simulink library "Lib_AP_Math"  (R2014b)
settings: Solver=ode45  StartTime=0.0  StopTime=10.0  RelTol=1e-3
settings Model: Creator=Ehang  LastModifiedBy=Ehang

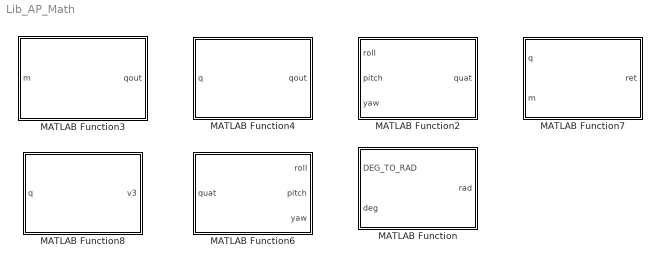
== system Lib_AP_Math ==
  MATLAB Function : MATLAB Function  TreatAsAtomicUnit=on
  MATLAB Function2 : MATLAB Function  TreatAsAtomicUnit=on
  MATLAB Function3 : MATLAB Function  TreatAsAtomicUnit=on
  MATLAB Function4 : MATLAB Function  TreatAsAtomicUnit=on
  MATLAB Function6 : MATLAB Function  TreatAsAtomicUnit=on
  MATLAB Function7 : MATLAB Function  TreatAsAtomicUnit=on
  MATLAB Function8 : MATLAB Function  TreatAsAtomicUnit=on

== matlab function Lib_AP_Math/MATLAB Function ==
  data: DEG_TO_RAD input; deg input; rad output
function rad = radians(DEG_TO_RAD,deg)
%#codegen
%将角度转化为弧度
rad = deg*DEG_TO_RAD;

== matlab function Lib_AP_Math/MATLAB Function2 ==
  data: roll input; pitch input; quat output; yaw input
function quat= from_euler(roll,pitch,yaw)
%%将欧拉角转化为四元数
%#codegen
    cr2 = cos(roll*0.5);
    cp2 = cos(pitch*0.5);
    cy2 = cos(yaw*0.5);
    sr2 = sin(roll*0.5);
    sp2 = sin(pitch*0.5);
    sy2 = sin(yaw*0.5);

    q1 = cr2*cp2*cy2 + sr2*sp2*sy2;
    q2 = sr2*cp2*cy2 - cr2*sp2*sy2;
    q3 = cr2*sp2*cy2 + sr2*cp2*sy2;
    q4 = cr2*cp2*sy2 - sr2*sp2*cy2;
    quat=[q1;q2;q3;q4];

% void Quaternion::from_euler(float roll, float pitch, float yaw)
% {
%     float cr2 = cosf(roll*0.5f);
%     float cp2 = cosf(pitch*0.5f);
%     float cy2 = cosf(yaw*0.5f);
%     float sr2 = sinf(roll*0.5f);
%     float sp2 = sinf(pitch*0.5f);
%     float sy2 = sinf(yaw*0.5f);
% 
%     q1 = cr2*cp2*cy2 + sr2*sp2*sy2;
%     q2 = sr2*cp2*cy2 - cr2*sp2*sy2;
%     q3 = cr2*sp2*cy2 + sr2*cp2*sy2;
%     q4 = cr2*cp2*sy2 - sr2*sp2*cy2;
% }

== matlab function Lib_AP_Math/MATLAB Function3 ==
  data: m input; qout output
function qout=from_rotation_matrix(m)
%#codegen
% //返回与旋转矩阵m等效的四元数qout
% // return the rotation matrix equivalent for this quaternion
% // Thanks to Martin John Baker
% // http://www.euclideanspace.com/maths/geometry/rotations/conversions/matrixToQuaternion/index.htm
%a,b,c是列数，x,y,z是行数
    m00 = m(1,1);
    m11 = m(2,2);
    m22 = m(3,3);
    m10 = m(1,2);
    m01 = m(2,1);
    m20 = m(1,3);
    m02 = m(3,1);
    m21 = m(2,3);
    m12 = m(3,2);
% m00 = m.a.x;
%     m11 = m.b.y;
%     m22 = m.c.z;
%     m10 = m.b.x;
%     m01 = m.a.y;
%     m20 = m.c.x;
%     m02 = m.a.z;
%     m21 = m.c.y;
%     m12 = m.b.z;
tr = m00 + m11 + m22;
%为什么有下划线 Matalb中elseif是连在一起的
    if (tr > 0) 
        S = sqrt(tr+1) * 2;
        qw = 0.25 * S;
        qx = (m21 - m12) / S;
        qy = (m02 - m20) / S;
        qz = (m10 - m01) / S;
    elseif (m00 > m11) && (m00 > m22) 
        S = sqrt(1.0 + m00 - m11 - m22) * 2;
        qw = (m21 - m12) / S;
        qx = 0.25 * S;
        qy = (m01 + m10) / S;
        qz = (m02 + m20) / S;
    elseif (m11 > m22) 
        S = sqrt(1.0+m11- m00 - m22) * 2;
        qw = (m02 - m20) / S;
        qx = (m01 + m10) / S;
        qy = 0.25* S;
        qz = (m12 + m21) / S;
    else 
        S = sqrt(1.0 + m22 - m00 - m11) * 2;
        qw = (m10 - m01) / S;
        qx = (m02 + m20) / S;
        qy = (m12 + m21) / S;
        qz = 0.25 * S;
    end
    qout=[qw;
          qx;
          qy;
          qz];

% // return the rotation matrix equivalent for this quaternion
% // Thanks to Martin John Baker
% // http://www.euclideanspace.com/maths/geometry/rotations/conversions/matrixToQuaternion/index.htm
% void Quaternion::from_rotation_matrix(const Matrix3f &m)
% {
%     const float &m00 = m.a.x;
%     const float &m11 = m.b.y;
%     const float &m22 = m.c.z;
%     const float &m10 = m.b.x;
%     const float &m01 = m.a.y;
%     const float &m20 = m.c.x;
%     const float &m02 = m.a.z;
%     const float &m21 = m.c.y;
%     const float &m12 = m.b.z;
%     float &qw = q1;
%     float &qx = q2;
%     float &qy = q3;
%     float &qz = q4;
% 
%     float tr = m00 + m11 + m22;
% 
%     if (tr > 0) {
%         float S = sqrtf(tr+1) * 2;
%         qw = 0.25f * S;
%         qx = (m21 - m12) / S;
%         qy = (m02 - m20) / S;
%         qz = (m10 - m01) / S;
%     } else if ((m00 > m11) && (m00 > m22)) {
%         float S = sqrtf(1.0f + m00 - m11 - m22) * 2;
%         qw = (m21 - m12) / S;
%         qx = 0.25f * S;
%         qy = (m01 + m10) / S;
%         qz = (m02 + m20) / S;
%     } else if (m11 > m22) {
%         float S = sqrtf(1.0f + m11 - m00 - m22) * 2;
%         qw = (m02 - m20) / S;
%         qx = (m01 + m10) / S;
%         qy = 0.25f * S;
%         qz = (m12 + m21) / S;
%     } else {
%         float S = sqrtf(1.0f + m22 - m00 - m11) * 2;
%         qw = (m10 - m01) / S;
%         qx = (m02 + m20) / S;
%         qy = (m12 + m21) / S;
%         qz = 0.25f * S;
%     }
% }

== matlab function Lib_AP_Math/MATLAB Function4 ==
  data: q input; qout output
function qout=inverse(q)
%#codegen
%四元素求逆
qout=[q(1), -q(2), -q(3), -q(4)]';
% Quaternion Quaternion::inverse(void) const
% {
%     return Quaternion(q1, -q2, -q3, -q4);
% }

== matlab function Lib_AP_Math/MATLAB Function6 ==
  data: roll output; pitch output; yaw output; quat input
function [roll,pitch,yaw]=to_euler(quat)
%将四元素转化为对应的欧拉角
%#codegen
q1=quat(1);
q2=quat(2);
q3=quat(3);
q4=quat(4);
 roll=(atan2(2.0*(q1*q2 + q3*q4), 1 - 2.0*(q2*q2 + q3*q3)));
 
 safe_asin=(2.0*(q1*q3 - q4*q2));
 %省略函数safe_asin
 pitch=asin(safe_asin);
 
yaw= atan2(2.0*(q1*q4 + q2*q3), 1 - 2.0*(q3*q3 + q4*q4));
%这个函数有待理论验证

== matlab function Lib_AP_Math/MATLAB Function7 ==
  data: q input; m input; ret output

%%%%%%%%%%%四元数乘法函数%%%%%%%%%%%%
% 只进行四元数乘法计算，不进行任何归一化处理
%调用举例
% % a=[1 2 2 3]';
% % b=[2 4 2 3]';
% % q=qmul(a,b)
function ret =qmul(q,m)
lm=q(1);
p1=q(2);
p2=q(3);
p3=q(4);
q1 =[lm -p1 -p2 -p3;
    p1  lm -p3  p2;
    p2  p3  lm -p1;
    p3 -p2  p1  lm]*m;
ret=q1;
% Quaternion ret;
%     const float &w1 = q1;
%     const float &x1 = q2;
%     const float &y1 = q3;
%     const float &z1 = q4;
% 
%     float w2 = v.q1;
%     float x2 = v.q2;
%     float y2 = v.q3;
%     float z2 = v.q4;
% 
%     ret.q1 = w1*w2 - x1*x2 - y1*y2 - z1*z2;
%     ret.q2 = w1*x2 + x1*w2 + y1*z2 - z1*y2;
%     ret.q3 = w1*y2 - x1*z2 + y1*w2 + z1*x2;
%     ret.q4 = w1*z2 + x1*y2 - y1*x2 + z1*w2;
% 
%     return ret;

== matlab function Lib_AP_Math/MATLAB Function8 ==
  data: q input; v3 output
function v3=to_axis_angle(q)
%#codegen
%四元数转化为对应的旋转矢量
v3=[q(2), q(3), q(4)]';
l=sqrt(q(2)*q(2)+q(3)*q(3)+q(4)*q(4));

if l>1.0e-12  %避免除以一个过小的数
    v3=v3/l;%转轴
    al=2.0*atan2(l,q(1));%旋转弧度
    v3=al*v3;
end
%
% float l = sqrt(sq(q2)+sq(q3)+sq(q4));
%     v = Vector3f(q2,q3,q4);
%     if (l >= 1.0e-12f) {
%         v /= l;
%         v *= wrap_PI(2.0f * atan2f(l,q1));
%     }
